simulink model "conti_ss_model"  (R2024b)
settings: Solver=VariableStepAuto  StartTime=0.0  StopTime=10.0  RelTol=1e-3
values from neighbouring files (symbols this model uses):
  A = [0,1; 0,-10]    [conti_ss_script.m]    (also in discrete_script.m = [0,1; -3, -60]; error_space_script.m = [0,1; 0,-20]; observer_script.m = [0,1; 0,-20]; pid_script.m)
  B = [0; 120]    [conti_ss_script.m]    (also in discrete_script.m = [0; 1]; error_space_script.m = [0; 60]; observer_script.m = [0; 60]; pid_script.m)
  K = Ke(2:end)    [conti_ss_script.m]    (also in discrete_script.m = Kdd; error_space_script.m = Kz(4:5); observer_script.m)
  Ki = Ke(1)    [conti_ss_script.m]    (also in observer_script.m; pid_script.m = -w_gc * dK*sin(dphi))
  nominal_robust = 1    [conti_ss_script.m]
  Nu = ff(3)    [conti_ss_script.m]    (also in discrete_script.m = Nudd; observer_script.m)
  Nx = ff(1:2)    [conti_ss_script.m]    (also in discrete_script.m = Nxdd; observer_script.m)
settings Model: Creator=pries  LastModifiedBy=pries

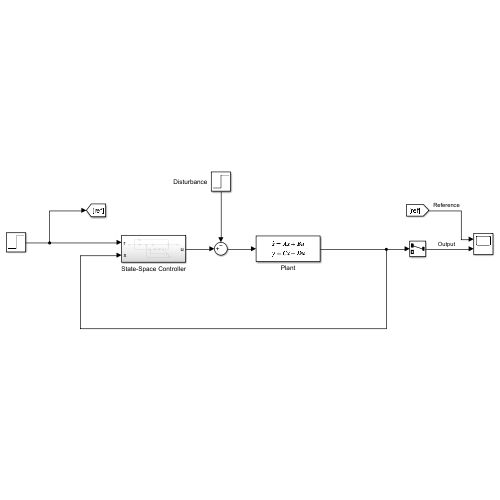
[thumbnail: Simulink's stored preview of the top-level diagram]
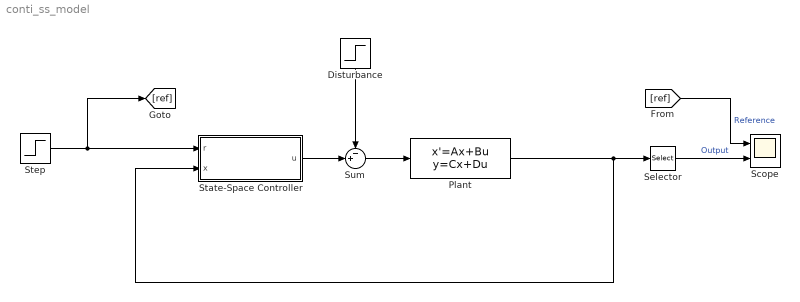
== system conti_ss_model ==
  Disturbance : Step  Time=3  SampleTime=0
  Plant : StateSpace  A=A  B=B  C=eye(2)  D=[0;0]  InitialCondition=0
  Scope : Scope  NumInputPorts=2
  Selector : Selector  InputPortWidth=2  IndexOptions=Index vector (dialog)  Indices=1  OutputSizes=1
  State-Space Controller : Subsystem
  Step : Step  Time=0  SampleTime=0
  Sum : Sum  Inputs=-+|
  wires:
  Step/1 -> State-Space Controller/1(r), [ref]
  Plant/1 -> State-Space Controller/2(x), Selector/1
  Selector/1 -> Scope/2  "Output"
  [ref] -> Scope/1  "Reference"
  Disturbance/1 -> Sum/1
  State-Space Controller/1(u) -> Sum/2
  Sum/1 -> Plant/1

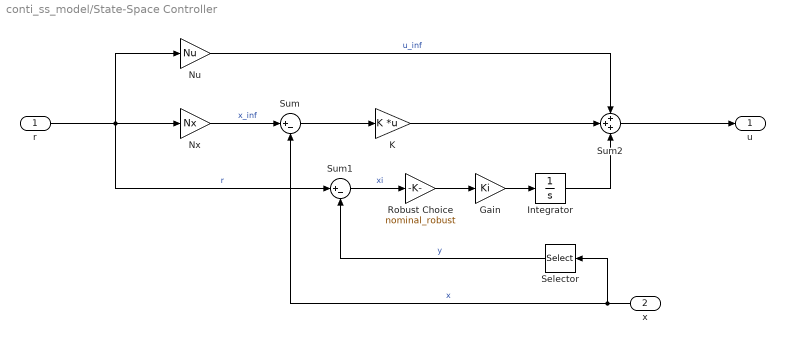
== system conti_ss_model/State-Space Controller ==
  r : Inport
  x : Inport  Port=2
  Gain : Gain  Gain=Ki
  Integrator : Integrator
  K : Gain  Gain=K  Multiplication=Matrix(K*u)
  Nu : Gain  Gain=Nu
  Nx : Gain  Gain=Nx
  Robust Choice : Gain  Gain=nominal_robust
  Selector : Selector  InputPortWidth=2  IndexOptions=Index vector (dialog)  Indices=1  OutputSizes=1
  Sum : Sum  Inputs=|+-
  Sum1 : Sum  Inputs=|+-
  Sum2 : Sum  Inputs=+++
  u : Outport
  wires:
  r/1 -> Sum1/1, Nu/1, Nx/1  "r"
  Nx/1 -> Sum/1  "x_inf"
  Sum/1 -> K/1
  x/1 -> Sum/2, Selector/1  "x"
  Selector/1 -> Sum1/2  "y"
  K/1 -> Sum2/2
  Nu/1 -> Sum2/1  "u_inf"
  Sum2/1 -> u/1
  Gain/1 -> Integrator/1
  Integrator/1 -> Sum2/3
  Robust Choice/1 -> Gain/1
  Sum1/1 -> Robust Choice/1  "xi"
